simulink model "pendulum_3a1"  (R2018b)
settings: Solver=VariableStepAuto  StartTime=0.0  StopTime=100  RelTol=1e-3
values from neighbouring files (symbols this model uses):
  A = [0 0 1 0;0 0 0 1;0 -Rod_m*g/Cart_m -(Kg^2)*Km*Kb/(Cart_m*Rm*motor_radius^2) 0 ... (first row only)    [pendulum_version1.m]
  B = [0;0;Km*Kg/(Cart_m*Rm*motor_radius);-Km*Kg/(Cart_m*Rm*motor_radius*Rod_l)]    [pendulum_version1.m]
  C = [1 0 0 0 ... (first row only)    [pendulum_version1.m]
  CC = [0.456/4.41 0; 0 90/6.328]    [pendulum_version1.m]
  D = [0 ... (first row only)    [pendulum_version1.m]
  K = lqr(A,B,Q,R)    [pendulum_version1.m]
  omega_c = 2*2*pi    (= 12.5663706144)    [pendulum_version1.m]
  Ts = 1/200    (= 0.005)    [pendulum_version1.m]
  xd = 2    [pendulum_version1.m]
libraries: simulink x1, simulink_extras x1
settings Model: Creator=paul-emileverleye  LastModifiedBy=Kyle
settings DebuggingCC: LibraryContextMissingDiagnostic=none
settings SFSimCC: SimUseLocalCustomCode=off
settings RTWCC: RTWUseLocalCustomCode=off

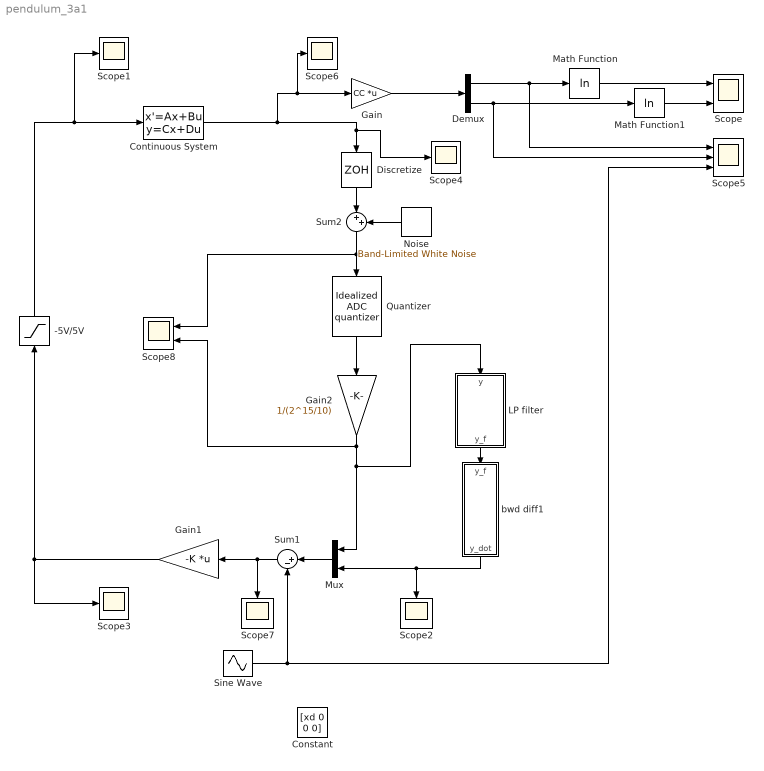
== system pendulum_3a1 ==
  -5V/5V : Saturate  UpperLimit=5  LowerLimit=-5
  Constant : Constant  Value=[xd 0 0 0]
  Continuous System : StateSpace  A=A  B=B  C=C  D=D  InitialCondition=0
  Demux : Demux  Outputs=2
  Discretize : ZeroOrderHold  SampleTime=1/200
  Gain : Gain  Gain=CC  Multiplication=Matrix(K*u)
  Gain1 : Gain  Gain=-K  Multiplication=Matrix(K*u)
  Gain2 : Gain  Gain=1/(2^15/10)
  LP filter : Subsystem
  Math Function : Math  Operator=log  OutputSignalType=real  SaturateOnIntegerOverflow=on
  Math Function1 : Math  Operator=log  OutputSignalType=real  SaturateOnIntegerOverflow=on
  Mux : Mux  Inputs=2
  Noise : simulink/Sources/Band-Limited White Noise  Cov=[0.0]  Ts=0.1  seed=[23341]
  Quantizer : simulink_extras/Additional Discrete/Idealized ADC quantizer  NumberOfConverterBits=16  Vmin=-10  Vmax=10  OutputDataType=double  OutputNegativeValues=on
      settings: SourceProductName=Simulink
  Scope : Scope  NumInputPorts=2
  Scope{1..4,6..7} (6 alike) : Scope
  Scope5 : Scope  NumInputPorts=3
  Scope8 : Scope  NumInputPorts=2
  Sine Wave : Sin  Amplitude=0.5  Frequency=0.2  SampleTime=0
  Sum1 : Sum  Inputs=|+-
  Sum2 : Sum  Inputs=|++
  bwd diff1 : Subsystem
  wires:
  Gain1/1 -> Scope3/1, -5V/5V/1
  -5V/5V/1 -> Continuous System/1, Scope1/1
  Demux/1 -> Scope5/1, Math Function/1
  Gain/1 -> Demux/1
  Demux/2 -> Scope5/2, Math Function1/1
  Sum1/1 -> Scope7/1, Gain1/1
  Continuous System/1 -> Scope6/1, Gain/1, Scope4/1, Discretize/1
  LP filter/1(y_f) -> bwd diff1/1(y_f)
  Noise/1 -> Sum2/2
  Discretize/1 -> Sum2/1
  Sum2/1 -> Scope8/1, Quantizer/1
  Mux/1 -> Sum1/1
  bwd diff1/1(y_dot) -> Mux/2, Scope2/1
  Math Function/1 -> Scope/1
  Math Function1/1 -> Scope/2
  Sine Wave/1 -> Sum1/2, Scope5/3
  Quantizer/1 -> Gain2/1
  Gain2/1 -> Scope8/2, LP filter/1(y), Mux/1

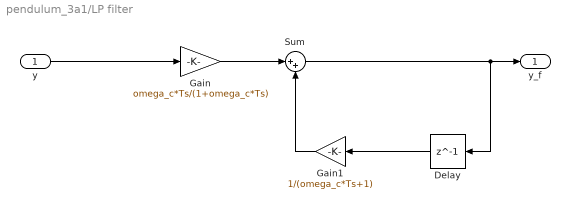
== system pendulum_3a1/LP filter ==
  y : Inport
  Delay : Delay  DelayLength=1  InitialCondition=0
  Gain : Gain  Gain=omega_c*Ts/(1+omega_c*Ts)
  Gain1 : Gain  Gain=1/(omega_c*Ts+1)
  Sum : Sum  Inputs=|++
  y_f : Outport
  wires:
  y/1 -> Gain/1
  Gain/1 -> Sum/1
  Delay/1 -> Gain1/1
  Gain1/1 -> Sum/2
  Sum/1 -> Delay/1, y_f/1

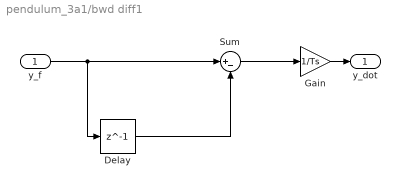
== system pendulum_3a1/bwd diff1 ==
  y_f : Inport
  Delay : Delay  DelayLength=1  InitialCondition=0
  Gain : Gain  Gain=1/Ts
  Sum : Sum  Inputs=|+-
  y_dot : Outport
  wires:
  y_f/1 -> Sum/1, Delay/1
  Gain/1 -> y_dot/1
  Delay/1 -> Sum/2
  Sum/1 -> Gain/1
